simulink subsystem "Guidance"  (R2023a)
settings: Solver=VariableStepAuto  StartTime=0.0  StopTime=10.0  RelTol=1e-3
values from neighbouring files (symbols this model uses):
  waypoint_struct = outWPS    [generating_waypoints.m]    (also in path_constructor.m)
libraries: uavalgslib x4, simulink x2
settings Model: Creator=jipva  LastModifiedBy=jipva

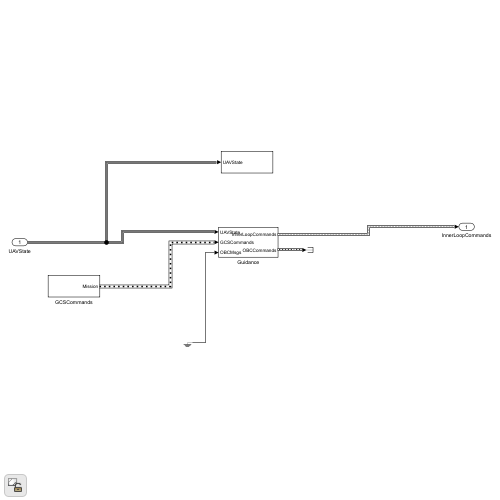
[thumbnail: Simulink's stored preview of the top-level diagram]
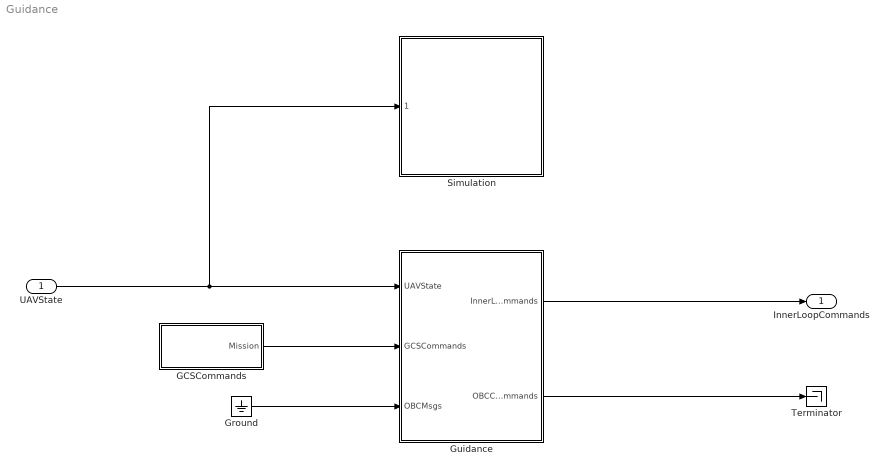
== system Guidance ==
  UAVState : Inport
  GCSCommands : Subsystem
  Ground : Ground
  Guidance : Subsystem
  Simulation : Subsystem  ReferencedSubsystem=Simulation
  Terminator : Terminator
  InnerLoopCommands : Outport
  wires:
  UAVState/1 -> Guidance/1(UAVState), Simulation/1
  GCSCommands/1(Mission) -> Guidance/2(GCSCommands)
  Ground/1 -> Guidance/3(OBCMsgs)
  Guidance/2(OBCCommands) -> Terminator/1
  Guidance/1(InnerLoopCommands) -> InnerLoopCommands/1

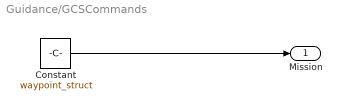
== system Guidance/GCSCommands ==
  Constant : Constant  Value=waypoint_struct  OutDataTypeStr=Bus: UAVPathManagerBus  SampleTime=-1
  Mission : Outport
  wires:
  Constant/1 -> Mission/1

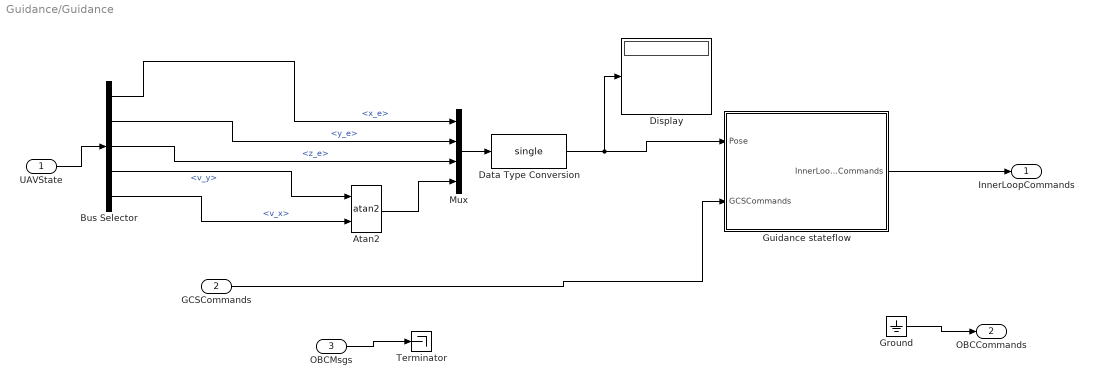
== system Guidance/Guidance ==
  UAVState : Inport
  GCSCommands : Inport  Port=2
  OBCMsgs : Inport  Port=3
  Atan2 : Trigonometry  Operator=atan2
  Bus Selector : BusSelector  OutputSignals=pos.x_e,pos.y_e,pos.z_e,V_e.v_y,V_e.v_x
  Data Type Conversion : DataTypeConversion  OutDataTypeStr=single  SaturateOnIntegerOverflow=off  RndMeth=Floor
  Display : Display
  Ground : Ground
  Guidance stateflow : Subsystem
  Mux : Mux
  Terminator : Terminator
  InnerLoopCommands : Outport
  OBCCommands : Outport  Port=2  OutDataTypeStr=Bus: UAVPathManagerBus
  wires:
  GCSCommands/1 -> Guidance stateflow/2(GCSCommands)
  Data Type Conversion/1 -> Guidance stateflow/1(Pose), Display/1
  Mux/1 -> Data Type Conversion/1
  Bus Selector/5 -> Atan2/2  "<v_x>"
  Bus Selector/4 -> Atan2/1  "<v_y>"
  Bus Selector/3 -> Mux/3  "<z_e>"
  Bus Selector/2 -> Mux/2  "<y_e>"
  Bus Selector/1 -> Mux/1  "<x_e>"
  UAVState/1 -> Bus Selector/1
  Ground/1 -> OBCCommands/1
  Guidance stateflow/1(InnerLoopCommands) -> InnerLoopCommands/1
  OBCMsgs/1 -> Terminator/1
  Atan2/1 -> Mux/4

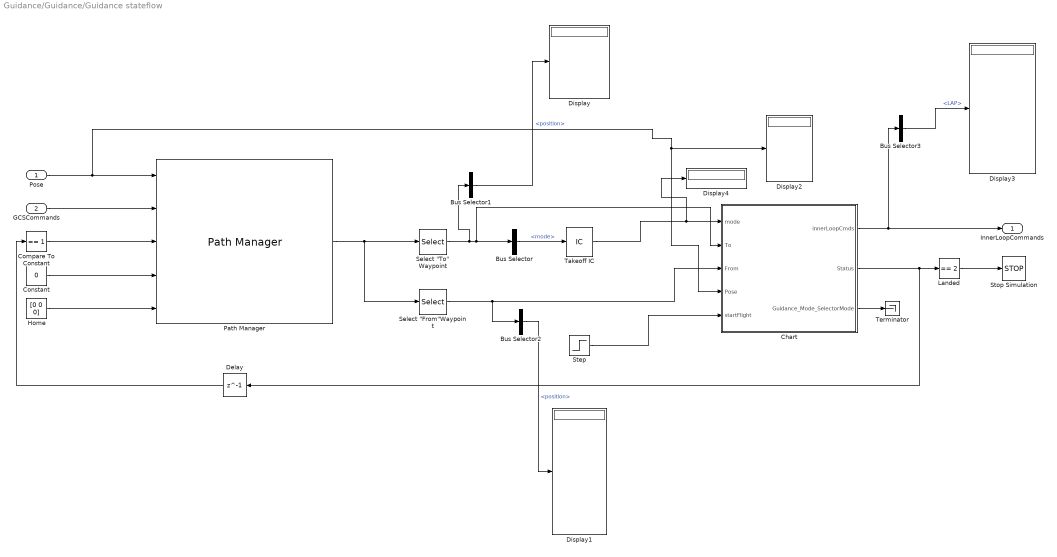
== system Guidance/Guidance/Guidance stateflow ==
  Pose : Inport
  GCSCommands : Inport  Port=2
  Bus Selector : BusSelector  OutputSignals=mode
  Bus Selector1 : BusSelector  OutputSignals=position
  Bus Selector2 : BusSelector  OutputSignals=position
  Bus Selector3 : BusSelector  OutputSignals=LAP
  Chart : Stateflow chart  TreatAsAtomicUnit=on
  Compare To Constant : simulink/Logic and Bit Operations/Compare To Constant  relop===  const=1  OutDataTypeStr=boolean
  Constant : Constant  Value=0  OutDataTypeStr=uint8
  Delay : Delay  DelayLength=1  InitialCondition=0
  Display{,1..4} (5 alike) : Display
  Home : Constant  Value=[0 0 0]  OutDataTypeStr=single
  Landed : simulink/Logic and Bit Operations/Compare To Constant  relop===  const=2  OutDataTypeStr=boolean
  Path Manager : uavalgslib/Path Manager  UAVType=multirotor  LoiterRadius=25  dataType=single  inputBusName='UAVPathManagerBus'  SimulateUsing=Code generation
  "Select \"From\"Waypoint" : Selector  InputPortWidth=2  IndexOptions=Index vector (dialog)  Indices=2  OutputSizes=1
  "Select \"To\" Waypoint" : Selector  InputPortWidth=2  IndexOptions=Index vector (dialog)  Indices=1  OutputSizes=1
  Step : Step  Time=0.5  SampleTime=0.02
  Stop Simulation : Stop
  Takeoff IC : InitialCondition
  Terminator : Terminator
  InnerLoopCommands : Outport  OutDataTypeStr=Bus: innerLoopCmdsBus
  wires:
  Bus Selector3/1 -> Display3/1  "<LAP>"
  Bus Selector2/1 -> Display1/1  "<position>"
  Bus Selector1/1 -> Display/1  "<position>"
  Chart/3(Guidance_Mode_SelectorMode) -> Terminator/1
  Takeoff IC/1 -> Chart/1(mode), Display4/1
  Chart/2(Status) -> Landed/1, Delay/1
  Chart/1(innerLoopCmds) -> InnerLoopCommands/1, Bus Selector3/1
  "Select \"From\"Waypoint"/1 -> Chart/3(From), Bus Selector2/1
  "Select \"To\" Waypoint"/1 -> Bus Selector/1, Chart/2(To), Bus Selector1/1
  Pose/1 -> Path Manager/1, Display2/1, Chart/4(Pose)
  Landed/1 -> Stop Simulation/1
  Step/1 -> Chart/5(startFlight)
  Compare To Constant/1 -> Path Manager/3
  Delay/1 -> Compare To Constant/1
  Bus Selector/1 -> Takeoff IC/1  "<mode>"
  Path Manager/1 -> "Select \"To\" Waypoint"/1, "Select \"From\"Waypoint"/1
  Constant/1 -> Path Manager/4
  Home/1 -> Path Manager/5
  GCSCommands/1 -> Path Manager/2

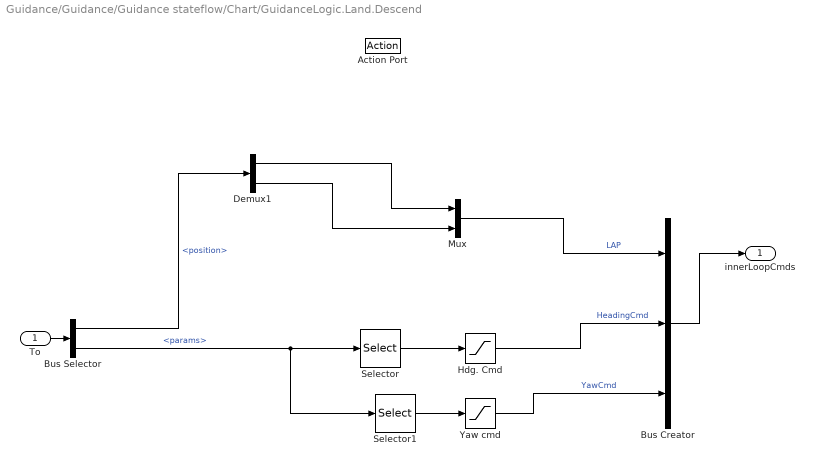
== system Guidance/Guidance/Guidance stateflow/Chart/GuidanceLogic.Land.Descend ==
  To : Inport
  Action Port : ActionPort
      settings: CopyFcn=Stateflow.SLINSF.SimulinkMan.removeBlockPreDeleteFcn  PreDeleteFcn=Stateflow.SLINSF.SimulinkMan.unsafePredeleteFcn
  Bus Creator : BusCreator  Inputs=3  OutDataTypeStr=Bus: innerLoopCmdsBus  NonVirtualBus=on
  Bus Selector : BusSelector  OutputSignals=position,params
  Demux1 : Demux  Outputs=[2 1]
  Hdg. Cmd : Saturate
  Mux : Mux  Inputs=2
  Selector : Selector  InputPortWidth=4  IndexOptions=Index vector (dialog)  Indices=4  OutputSizes=1
  Selector1 : Selector  InputPortWidth=4  IndexOptions=Index vector (dialog)  Indices=4  OutputSizes=1
  Yaw cmd : Saturate  UpperLimit=pi  LowerLimit=-pi
  innerLoopCmds : Outport  OutDataTypeStr=Bus: innerLoopCmdsBus
  wires:
  To/1 -> Bus Selector/1
  Bus Creator/1 -> innerLoopCmds/1
  Yaw cmd/1 -> Bus Creator/3  "YawCmd"
  Selector/1 -> Hdg. Cmd/1
  Hdg. Cmd/1 -> Bus Creator/2  "HeadingCmd"
  Demux1/1 -> Mux/1
  Selector1/1 -> Yaw cmd/1
  Bus Selector/2 -> Selector/1, Selector1/1  "<params>"
  Mux/1 -> Bus Creator/1  "LAP"
  Demux1/2 -> Mux/2
  Bus Selector/1 -> Demux1/1  "<position>"

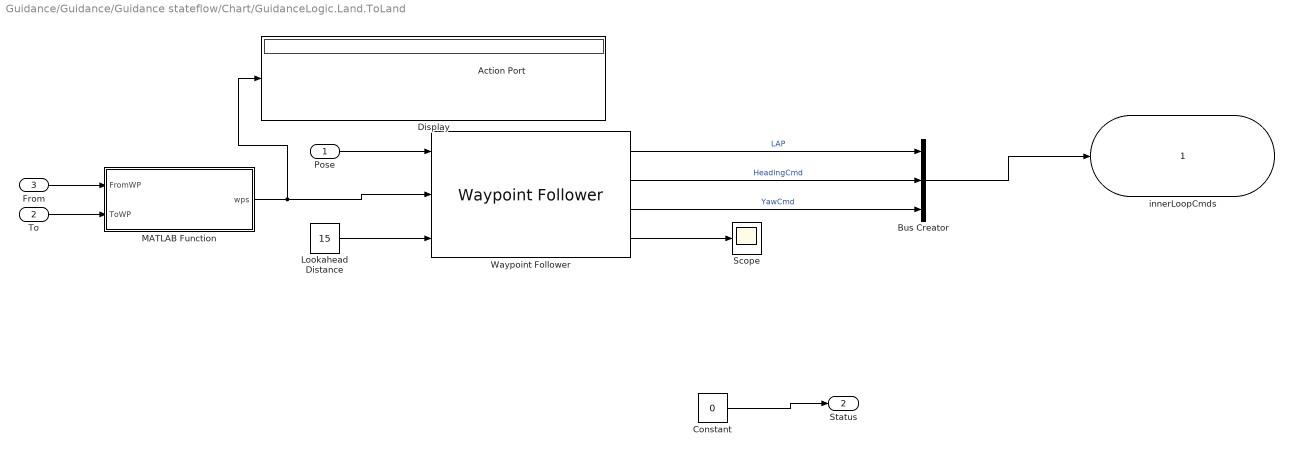
== system Guidance/Guidance/Guidance stateflow/Chart/GuidanceLogic.Land.ToLand ==
  Pose : Inport
  To : Inport  Port=2
  From : Inport  Port=3
  Action Port : ActionPort
      settings: CopyFcn=Stateflow.SLINSF.SimulinkMan.removeBlockPreDeleteFcn  PreDeleteFcn=Stateflow.SLINSF.SimulinkMan.unsafePredeleteFcn
  Bus Creator : BusCreator  Inputs=3  OutDataTypeStr=Bus: innerLoopCmdsBus  NonVirtualBus=on
  Constant : Constant  Value=0  OutDataTypeStr=uint8
  Display : Display
  Lookahead Distance : Constant  Value=15  OutDataTypeStr=single
  MATLAB Function : MATLAB Function  TreatAsAtomicUnit=on
  Scope : Scope
  Waypoint Follower : uavalgslib/Waypoint Follower  UAVType=multirotor  StartFrom=first  TransitionRadiusSource=internal  TransitionRadius=10  MinLookaheadDistance=0.1  YawInput=on  ShowCrossTrackErrorOutput=off  ShowStatusOutput=off  SimulateUsing=Interpreted execution
  innerLoopCmds : Outport  OutDataTypeStr=Bus: innerLoopCmdsBus
  Status : Outport  Port=2
  wires:
  Constant/1 -> Status/1
  Waypoint Follower/3 -> Bus Creator/3  "YawCmd"
  Lookahead Distance/1 -> Waypoint Follower/3
  Waypoint Follower/4 -> Scope/1
  Waypoint Follower/2 -> Bus Creator/2  "HeadingCmd"
  Pose/1 -> Waypoint Follower/1
  From/1 -> MATLAB Function/1(FromWP)
  Bus Creator/1 -> innerLoopCmds/1
  Waypoint Follower/1 -> Bus Creator/1  "LAP"
  MATLAB Function/1(wps) -> Waypoint Follower/2, Display/1
  To/1 -> MATLAB Function/2(ToWP)

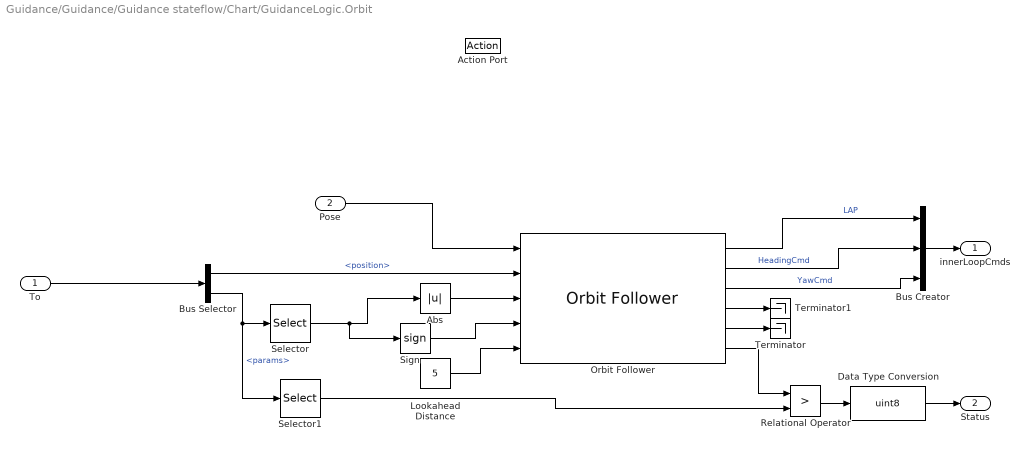
== system Guidance/Guidance/Guidance stateflow/Chart/GuidanceLogic.Orbit ==
  To : Inport
  Pose : Inport  Port=2
  Action Port : ActionPort
      settings: CopyFcn=Stateflow.SLINSF.SimulinkMan.removeBlockPreDeleteFcn  PreDeleteFcn=Stateflow.SLINSF.SimulinkMan.unsafePredeleteFcn
  Abs : Abs  SaturateOnIntegerOverflow=off
  Bus Creator : BusCreator  Inputs=3  OutDataTypeStr=Bus: innerLoopCmdsBus  NonVirtualBus=on
  Bus Selector : BusSelector  OutputSignals=position,params
  Data Type Conversion : DataTypeConversion  OutDataTypeStr=uint8  SaturateOnIntegerOverflow=off  RndMeth=Floor
  Lookahead Distance : Constant  Value=5  OutDataTypeStr=single
  Orbit Follower : uavalgslib/Orbit Follower  UAVType=multirotor  MinOrbitRadius=1  MinLookaheadDistance=0.1  ExternalReset=none  ShowCrossTrackErrorOutput=off  ShowNumTurnsOutput=on  SimulateUsing=Code generation
  Relational Operator : RelationalOperator  Operator=>  OutDataTypeStr=boolean  RndMeth=Simplest  InputSameDT=off
  Selector : Selector  InputPortWidth=4  IndexOptions=Index vector (dialog)  Indices=[3]  OutputSizes=1
  Selector1 : Selector  InputPortWidth=4  IndexOptions=Index vector (dialog)  Indices=[1]  OutputSizes=1
  Sign : Signum
  Terminator : Terminator
  Terminator1 : Terminator
  innerLoopCmds : Outport  OutDataTypeStr=Bus: innerLoopCmdsBus
  Status : Outport  Port=2
  wires:
  Data Type Conversion/1 -> Status/1
  Relational Operator/1 -> Data Type Conversion/1
  Selector1/1 -> Relational Operator/2
  Orbit Follower/6 -> Relational Operator/1
  Sign/1 -> Orbit Follower/4
  Lookahead Distance/1 -> Orbit Follower/5
  Selector/1 -> Abs/1, Sign/1
  Abs/1 -> Orbit Follower/3
  Bus Selector/2 -> Selector/1, Selector1/1  "<params>"
  Bus Selector/1 -> Orbit Follower/2  "<position>"
  Pose/1 -> Orbit Follower/1
  Bus Creator/1 -> innerLoopCmds/1
  Orbit Follower/3 -> Bus Creator/3  "YawCmd"
  Orbit Follower/2 -> Bus Creator/2  "HeadingCmd"
  Orbit Follower/1 -> Bus Creator/1  "LAP"
  Orbit Follower/5 -> Terminator/1
  Orbit Follower/4 -> Terminator1/1
  To/1 -> Bus Selector/1

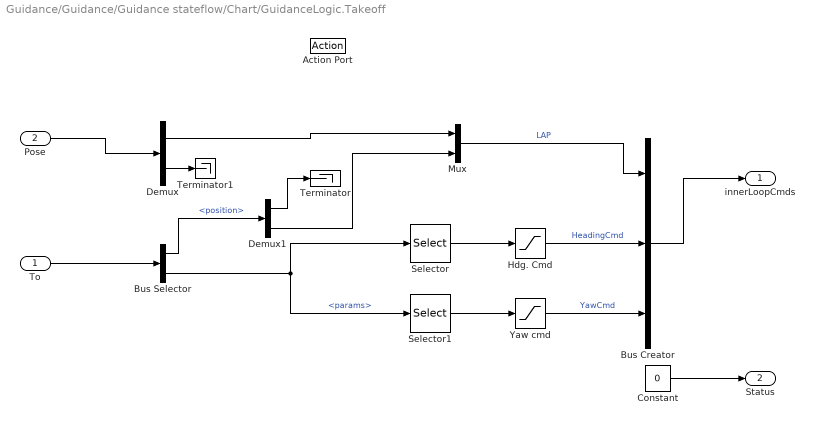
== system Guidance/Guidance/Guidance stateflow/Chart/GuidanceLogic.Takeoff ==
  To : Inport
  Pose : Inport  Port=2
  Action Port : ActionPort
      settings: CopyFcn=Stateflow.SLINSF.SimulinkMan.removeBlockPreDeleteFcn  PreDeleteFcn=Stateflow.SLINSF.SimulinkMan.unsafePredeleteFcn
  Bus Creator : BusCreator  Inputs=3  OutDataTypeStr=Bus: innerLoopCmdsBus  NonVirtualBus=on
  Bus Selector : BusSelector  OutputSignals=position,params
  Constant : Constant  Value=0  OutDataTypeStr=uint8
  Demux : Demux  Outputs=[2 2]
  Demux1 : Demux  Outputs=2
  Hdg. Cmd : Saturate
  Mux : Mux  Inputs=2
  Selector : Selector  InputPortWidth=4  IndexOptions=Index vector (dialog)  Indices=4  OutputSizes=1
  Selector1 : Selector  InputPortWidth=4  IndexOptions=Index vector (dialog)  Indices=4  OutputSizes=1
  Terminator : Terminator
  Terminator1 : Terminator
  Yaw cmd : Saturate  UpperLimit=pi  LowerLimit=-pi
  innerLoopCmds : Outport  OutDataTypeStr=Bus: innerLoopCmdsBus
  Status : Outport  Port=2
  wires:
  Constant/1 -> Status/1
  Yaw cmd/1 -> Bus Creator/3  "YawCmd"
  Selector/1 -> Hdg. Cmd/1
  Selector1/1 -> Yaw cmd/1
  Hdg. Cmd/1 -> Bus Creator/2  "HeadingCmd"
  Demux/2 -> Terminator1/1
  Bus Creator/1 -> innerLoopCmds/1
  Bus Selector/2 -> Selector/1, Selector1/1  "<params>"
  Demux1/2 -> Mux/2
  Demux1/1 -> Terminator/1
  Bus Selector/1 -> Demux1/1  "<position>"
  To/1 -> Bus Selector/1
  Mux/1 -> Bus Creator/1  "LAP"
  Demux/1 -> Mux/1
  Pose/1 -> Demux/1

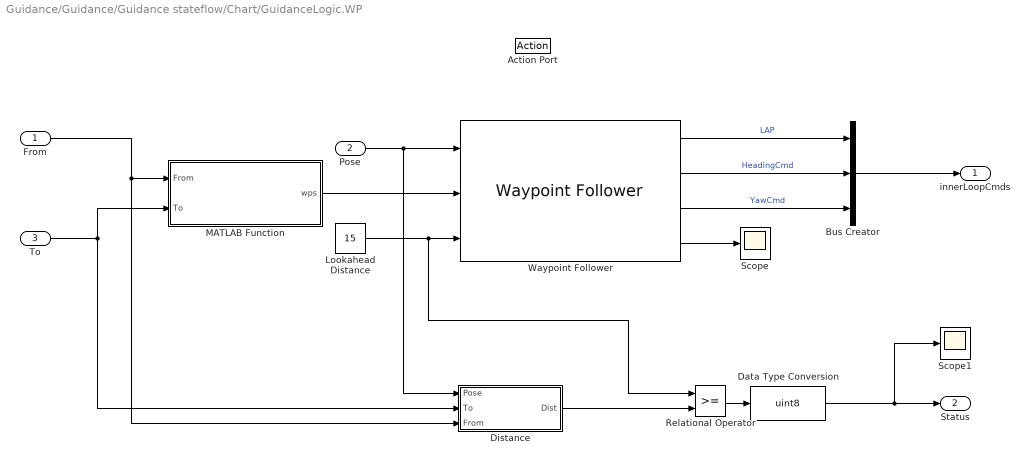
== system Guidance/Guidance/Guidance stateflow/Chart/GuidanceLogic.WP ==
  From : Inport
  Pose : Inport  Port=2
  To : Inport  Port=3
  Action Port : ActionPort
      settings: CopyFcn=Stateflow.SLINSF.SimulinkMan.removeBlockPreDeleteFcn  PreDeleteFcn=Stateflow.SLINSF.SimulinkMan.unsafePredeleteFcn
  Bus Creator : BusCreator  Inputs=3  OutDataTypeStr=Bus: innerLoopCmdsBus  NonVirtualBus=on
  Data Type Conversion : DataTypeConversion  OutDataTypeStr=uint8  SaturateOnIntegerOverflow=off  RndMeth=Floor
  Distance : Subsystem
  Lookahead Distance : Constant  Value=15  OutDataTypeStr=single
  MATLAB Function : MATLAB Function  TreatAsAtomicUnit=on
  Relational Operator : RelationalOperator  OutDataTypeStr=boolean  RndMeth=Simplest  InputSameDT=off
  Scope : Scope
  Scope1 : Scope
  Waypoint Follower : uavalgslib/Waypoint Follower  UAVType=multirotor  StartFrom=first  TransitionRadiusSource=internal  TransitionRadius=10  MinLookaheadDistance=0.1  YawInput=on  ShowCrossTrackErrorOutput=off  ShowStatusOutput=off  SimulateUsing=Code generation
  innerLoopCmds : Outport  OutDataTypeStr=Bus: innerLoopCmdsBus
  Status : Outport  Port=2
  wires:
  Waypoint Follower/3 -> Bus Creator/3  "YawCmd"
  Lookahead Distance/1 -> Waypoint Follower/3, Relational Operator/1
  Distance/1(Dist) -> Relational Operator/2
  Relational Operator/1 -> Data Type Conversion/1
  Waypoint Follower/4 -> Scope/1
  Waypoint Follower/2 -> Bus Creator/2  "HeadingCmd"
  Pose/1 -> Waypoint Follower/1, Distance/1(Pose)
  From/1 -> MATLAB Function/1(From), Distance/3(From)
  Bus Creator/1 -> innerLoopCmds/1
  Data Type Conversion/1 -> Status/1, Scope1/1
  Waypoint Follower/1 -> Bus Creator/1  "LAP"
  MATLAB Function/1(wps) -> Waypoint Follower/2
  To/1 -> Distance/2(To), MATLAB Function/2(To)

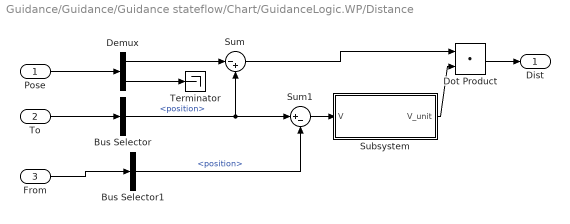
== system Guidance/Guidance/Guidance stateflow/Chart/GuidanceLogic.WP/Distance ==
  Pose : Inport
  To : Inport  Port=2
  From : Inport  Port=3
  Bus Selector : BusSelector  OutputSignals=position
  Bus Selector1 : BusSelector  OutputSignals=position
  Demux : Demux  Outputs=[3 1]
  Dot Product : DotProduct  OutDataTypeStr=Inherit: Inherit via internal rule
  Subsystem : Subsystem
  Sum : Sum  Inputs=|-+
  Sum1 : Sum  Inputs=|+-
  Terminator : Terminator
  Dist : Outport
  wires:
  Subsystem/1(V_unit) -> Dot Product/2
  Sum1/1 -> Subsystem/1(V)
  Dot Product/1 -> Dist/1
  Sum/1 -> Dot Product/1
  Bus Selector/1 -> Sum1/1, Sum/2  "<position>"
  Bus Selector1/1 -> Sum1/2  "<position>"
  From/1 -> Bus Selector1/1
  To/1 -> Bus Selector/1
  Demux/2 -> Terminator/1
  Demux/1 -> Sum/1
  Pose/1 -> Demux/1

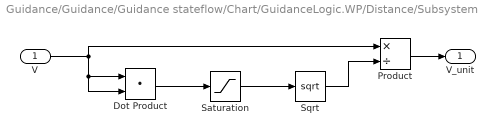
== system Guidance/Guidance/Guidance stateflow/Chart/GuidanceLogic.WP/Distance/Subsystem ==
  V : Inport
  Dot Product : DotProduct  OutDataTypeStr=Inherit: Inherit via internal rule
  Product : Product  Inputs=*/
  Saturation : Saturate
  Sqrt : Sqrt
  V_unit : Outport
  wires:
  Sqrt/1 -> Product/2
  Product/1 -> V_unit/1
  V/1 -> Product/1, Dot Product/2, Dot Product/1
  Saturation/1 -> Sqrt/1
  Dot Product/1 -> Saturation/1

== matlab function Guidance/Guidance stateflow/Chart/GuidanceLogic.WP/MATLAB Function ==
  data: From input Bus: UAVPathManagerBus; wps output; To input Bus: UAVPathManagerBus
function wps = getWaypointMission(From, To)

persistent outWPS

if isempty(outWPS)
    outWPS = single(zeros(2,4));
end

outWPS(1,:) = [From.position' From.params(4)];
outWPS(2,:) = [To.position' To.params(4)];

% for ii=1:2
%     outWPS(ii,1:3) = GCSMission(ii).position';
%     outWPS(ii,4) = GCSMission(ii).params(4);
% end

wps = outWPS;

== stateflow chart Guidance/Guidance stateflow/Chart ==
  settings: updateMethod=DISCRETE  sampleTime=0.02
  state GuidanceLogic
    state OnGround
    state Takeoff
    state WP
    state Orbit
    state Land
      state ToLand
      state Descend
      (default) -> ToLand
      ToLand -> Descend
    (default) -> OnGround
    OnGround -> (junction 12) : [startFlight == 1]
    GuidanceLogic -> (junction 12) : [hasChanged(mode)]
    (junction 12) -> Takeoff [order 1] : [mode == 1]
    (junction 12) -> (junction 10) [order 2]
    Takeoff -> WP : [Pose(3) <= To.position(3)]{Status = 1;}
    (junction 10) -> WP [order 1] : [mode == 2]
    (junction 10) -> (junction 11) [order 2]
    (junction 11) -> Orbit [order 1] : [mode == 3]
    (junction 11) -> (junction 29) [order 2]
    (junction 29) -> Land
    Land -> GuidanceLogic : [Pose(3)>=-0.1]{Status = 2;}
  (default) -> GuidanceLogic
  data: sf_internal_action_state_placeholder_data local double size=1 =0; sf_internal_action_state_placeholder_data local double size=1 =0; sf_internal_action_state_placeholder_data local double size=1 =0; sf_internal_action_state_placeholder_data local double size=1 =0; sf_internal_action_state_placeholder_data local double size=1 =0; innerLoopCmds output Bus: innerLoopCmdsBus; Status output uint8; mode input; To input Bus: UAVPathManagerBus; From input Bus: UAVPathManagerBus; Pose input; startFlight input; Guidance_Mode_SelectorMode output Enum: Guidance_Mode_SelectorModeType

== matlab function Guidance/Guidance stateflow/Chart/GuidanceLogic.Land.ToLand/MATLAB Function ==
  data: FromWP input; wps output; ToWP input
function wps = getLandingWaypoint(FromWP, ToWP)

persistent outWPS

if isempty(outWPS)
    outWPS = single(zeros(2,4));
end

outWPS(1,:) = [FromWP.position' FromWP.params(4)];
outWPS(2,:) = [ToWP.position(1:2)' FromWP.position(3) ToWP.params(4)];

wps = outWPS;
